simulink model "DockingApproachExample_Ext"  (Simulink 8.7)
settings: Solver=FixedStepDiscrete  StartTime=0.0  StopTime=300  RelTol=1e-3
model workspace (MAT data in the model file):
  input_struct.time = [0; 1; 2; 3; 4; 5; 6; 7; 8; 9; 10; 11; 12; 13; 14; 15; 16; 17; 18; 19; 20; 21; 22; 23; 24; 25; 26; 27; 28; 29; 30; 31; 32; 33; 34; 35; 36; 37; 38; 39; 40; 41; 42; 43; 44; 45; 46; 47; 48; 49; 50; 51; 52; 53; 54; 55; 56; 57; 58; 59; 60; 61; 62; 63; 64; 65; 66; 67; 68; 69; 70; 71; 72; 73; 74; 75; 76; 77; 78; 79; 80; 81; 82; 83; 84; 85; 86; 87; 88; 89; 90; 91; 92; 93; 94; 95; 96; 97; 98; 99; 100]
  input_struct.signals(1).name = 'GroundTrack_OrbitalPosition'
  input_struct.signals(1).values = [82; 91; 13; 92; 64; 10; 28; 55; 96; 97; 16; 98; 96; 49; 81; 15; 43; 92; 80; 96; 66; 4; 85; 94; 68; 76; 75; 40; 66; 18; 71; 4; 28; 5; 10; 83; 70; 32; 96; 4; 44; 39; 77; 80; 19; 49; 45; 65; 71; 76; 28; 68; 66; 17; 12; 50; 96; 35; 59; 23; 76; 26; 51; 70; 90; 96; 55; 14; 15; 26; 85; 26; 82; 25; 93; 35; 20; 26; 62; 48; 36; 84; 59; 55; 92; 29; 76; 76; 39; 57; 8; 6; 54; 78; 94; 13; 57; 47; 2; 34; 17]
  input_struct.signals(1).dimensions = 1
  input_struct.signals(2).name = 'GroundTrack_OrbitalVelocity'
  input_struct.signals(2).values = [80; 32; 53; 17; 61; 27; 66; 69; 75; 46; 9; 23; 92; 16; 83; 54; 100; 8; 45; 11; 97; 1; 78; 82; 87; 9; 40; 26; 81; 44; 92; 19; 27; 15; 14; 87; 58; 55; 15; 86; 63; 36; 52; 41; 8; 24; 13; 19; 24; 42; 5; 91; 95; 50; 49; 34; 91; 37; 12; 79; 39; 25; 41; 10; 14; 95; 96; 58; 6; 24; 36; 83; 2; 5; 17; 65; 74; 65; 46; 55; 30; 75; 19; 69; 19; 37; 63; 79; 9; 93; 78; 49; 44; 45; 31; 51; 52; 82; 80; 65; 38]
  input_struct.signals(2).dimensions = 1
  input_struct.signals(3).name = 'dockVisibility_status'
  input_struct.signals(3).values = [82; 54; 36; 94; 88; 56; 63; 59; 21; 31; 48; 24; 85; 20; 23; 18; 23; 44; 32; 93; 44; 19; 91; 98; 44; 12; 26; 41; 60; 27; 61; 72; 23; 12; 30; 32; 43; 51; 9; 27; 81; 3; 93; 74; 49; 58; 24; 46; 97; 55; 53; 24; 49; 63; 68; 40; 37; 99; 4; 89; 92; 80; 10; 27; 34; 68; 14; 73; 11; 66; 50; 78; 72; 91; 90; 34; 70; 20; 4; 75; 51; 48; 91; 61; 62; 86; 81; 58; 19; 24; 89; 3; 49; 17; 98; 72; 51; 48; 6; 69; 5]
  input_struct.signals(3).dimensions = 1
  input_struct.signals(4).name = 'opticsAvailability_status'
  input_struct.signals(4).values = [1; 1; 1; 1; 1; 1; 1; 1; 1; 1; 1; 1; 1; 1; 1; 1; 1; 1; 1; 1; 1; 1; 1; 1; 1; 1; 1; 1; 1; 1; 1; 1; 1; 1; 1; 1; 1; 1; 1; 1; 1; 1; 1; 1; 1; 1; 1; 1; 1; 1; 1; 1; 1; 1; 1; 1; 1; 1; 1; 1; 1; 1; 1; 1; 1; 1; 1; 1; 1; 1; 1; 1; 1; 1; 1; 1; 1; 1; 1; 1; 1; 1; 1; 1; 1; 1; 1; 1; 1; 1; 1; 1; 1; 1; 1; 1; 1; 1; 1; 1; 1]
  input_struct.signals(4).dimensions = 1
  input_struct.signals(5).name = 'sunlight_status'
  input_struct.signals(5).values = [1; 1; 1; 1; 1; 1; 1; 1; 1; 1; 1; 1; 1; 1; 1; 1; 1; 1; 1; 1; 1; 1; 1; 1; 1; 1; 1; 1; 1; 1; 1; 1; 1; 1; 1; 1; 1; 1; 1; 1; 1; 1; 1; 1; 1; 1; 1; 1; 1; 1; 1; 1; 1; 1; 1; 1; 1; 1; 1; 1; 1; 1; 1; 1; 1; 1; 1; 1; 1; 1; 1; 1; 1; 1; 1; 1; 1; 1; 1; 1; 1; 1; 1; 1; 1; 1; 1; 1; 1; 1; 1; 1; 1; 1; 1; 1; 1; 1; 1; 1; 1]
  input_struct.signals(5).dimensions = 1
  input_struct.signals(6).name = 'GPS_satelliteVisibility_status'
  input_struct.signals(6).values = [12; 94; 65; 48; 64; 55; 65; 55; 73; 53; 100; 22; 11; 11; 7; 41; 45; 37; 77; 63; 78; 94; 98; 20; 14; 70; 10; 53; 54; 87; 49; 40; 68; 75; 53; 35; 15; 59; 27; 5; 76; 25; 45; 69; 36; 74; 40; 69; 71; 45; 2; 34; 43; 28; 20; 83; 43; 89; 40; 77; 40; 81; 76; 38; 22; 80; 95; 33; 68; 44; 84; 77; 17; 87; 99; 52; 89; 59; 16; 20; 41; 75; 83; 79; 32; 54; 9; 12; 14; 68; 50; 19; 50; 15; 6; 86; 57; 93; 70; 59; 82]
  input_struct.signals(6).dimensions = 1
  input_struct.signals(7).name = 'GPS_receiverAvailability_status'
  input_struct.signals(7).values = [1; 1; 1; 1; 1; 1; 1; 1; 1; 1; 1; 1; 1; 1; 1; 1; 1; 1; 1; 1; 1; 1; 1; 1; 1; 1; 1; 1; 1; 1; 1; 1; 1; 1; 1; 1; 1; 1; 1; 1; 1; 1; 1; 1; 1; 1; 1; 1; 1; 1; 1; 1; 1; 1; 1; 1; 1; 1; 1; 1; 1; 1; 1; 1; 1; 1; 1; 1; 1; 1; 1; 1; 1; 1; 1; 1; 1; 1; 1; 1; 1; 1; 1; 1; 1; 1; 1; 1; 1; 1; 1; 1; 1; 1; 1; 1; 1; 1; 1; 1; 1]
  input_struct.signals(7).dimensions = 1
  input_struct.signals(8).name = 'StarPlanetTracker_planetVisibility'
  input_struct.signals(8).values = [34; 90; 12; 99; 54; 71; 100; 29; 42; 47; 77; 82; 11; 18; 36; 6; 53; 34; 18; 21; 91; 68; 47; 92; 11; 75; 74; 57; 19; 60; 30; 14; 22; 90; 8; 25; 6; 45; 2; 90; 20; 10; 31; 46; 11; 100; 34; 30; 7; 30; 5; 51; 77; 64; 9; 9; 78; 91; 54; 11; 83; 34; 30; 75; 2; 5; 67; 61; 53; 73; 71; 79; 29; 70; 56; 40; 7; 79; 34; 61; 75; 11; 13; 55; 49; 90; 80; 74; 6; 8; 9; 80; 95; 69; 14; 73; 12; 12; 65; 33; 66]
  input_struct.signals(8).dimensions = 1
  input_struct.signals(9).name = 'StarPlanetTracker_starVisibility'
  input_struct.signals(9).values = [75; 59; 75; 24; 74; 98; 87; 9; 37; 37; 69; 60; 79; 37; 21; 9; 78; 21; 39; 56; 23; 65; 49; 16; 79; 11; 30; 24; 54; 10; 41; 11; 12; 79; 30; 61; 97; 44; 70; 76; 44; 66; 11; 94; 19; 27; 80; 49; 77; 40; 28; 4; 68; 43; 46; 61; 6; 32; 78; 70; 13; 14; 10; 1; 43; 66; 73; 54; 11; 64; 13; 14; 10; 15; 17; 20; 32; 32; 22; 26; 90; 71; 56; 19; 22; 8; 92; 71; 56; 32; 17; 63; 99; 18; 26; 40; 8; 69; 41; 99; 41]
  input_struct.signals(9).dimensions = 1
  input_struct.signals(10).name = 'InertialNavigation_time'
  input_struct.signals(10).values = [1; 1; 1; 1; 1; 1; 1; 1; 1; 1; 1; 1; 1; 1; 1; 1; 1; 1; 1; 1; 1; 1; 1; 1; 1; 1; 1; 1; 1; 1; 1; 1; 1; 1; 1; 1; 1; 1; 1; 1; 1; 1; 1; 1; 1; 1; 1; 1; 1; 1; 1; 1; 1; 1; 1; 1; 1; 1; 1; 1; 1; 1; 1; 1; 1; 1; 1; 1; 1; 1; 1; 1; 1; 1; 1; 1; 1; 1; 1; 1; 1; 1; 1; 1; 1; 1; 1; 1; 1; 1; 1; 1; 1; 1; 1; 1; 1; 1; 1; 1; 1]
  input_struct.signals(10).dimensions = 1
  input_struct.signals(11).name = 'GroundTrack_Time'
  input_struct.signals(11).values = [19; 73; 38; 85; 74; 58; 18; 96; 27; 93; 23; 38; 9; 65; 19; 5; 73; 35; 67; 39; 63; 3; 92; 81; 75; 82; 39; 62; 58; 54; 28; 25; 46; 23; 81; 99; 3; 54; 9; 81; 99; 7; 94; 2; 69; 79; 54; 89; 90; 63; 14; 22; 19; 5; 11; 62; 94; 36; 42; 99; 95; 68; 99; 77; 34; 67; 25; 30; 69; 53; 42; 61; 76; 59; 56; 59; 52; 9; 72; 100; 36; 98; 35; 89; 46; 42; 22; 13; 31; 73; 79; 70; 1; 85; 93; 78; 5; 38; 71; 73; 23]
  input_struct.signals(11).dimensions = 1
  input_struct.signals(12).name = 'RealTimeClock_time'
  input_struct.signals(12).values = [27; 68; 48; 63; 24; 18; 83; 77; 94; 11; 19; 10; 49; 20; 90; 10; 5; 56; 78; 32; 18; 34; 22; 52; 91; 63; 11; 40; 6; 51; 44; 100; 82; 49; 90; 14; 40; 93; 92; 72; 62; 35; 94; 13; 74; 65; 84; 40; 75; 84; 33; 56; 98; 55; 34; 62; 37; 76; 42; 50; 70; 98; 33; 84; 74; 96; 4; 36; 67; 29; 24; 72; 63; 60; 67; 5; 35; 46; 25; 72; 86; 29; 74; 14; 84; 14; 59; 37; 81; 51; 49; 88; 36; 45; 97; 5; 98; 19; 67; 59; 68]
  input_struct.signals(12).dimensions = 1
  input_struct.signals(13).name = 'StageTransition'
  input_struct.signals(13).values = [37; 63; 82; 2; 9; 98; 66; 24; 41; 13; 27; 26; 34; 16; 35; 13; 89; 10; 94; 40; 5; 35; 74; 80; 55; 69; 90; 6; 31; 5; 20; 73; 73; 88; 59; 8; 93; 81; 29; 55; 99; 72; 84; 44; 48; 57; 27; 75; 51; 65; 31; 14; 48; 37; 79; 79; 67; 14; 3; 56; 31; 94; 99; 29; 81; 90; 60; 89; 95; 55; 73; 58; 3; 45; 65; 53; 38; 94; 83; 85; 38; 60; 88; 94; 67; 21; 66; 8; 41; 67; 94; 82; 49; 76; 42; 98; 99; 87; 39; 46; 25]
  input_struct.signals(13).dimensions : numeric (value not decoded)
libraries: simulink x11
(part 1 of 2)
settings Model: Creator=mwwhalen  LastModifiedBy=bourbouh
settings DataIOCC: ExternalInput=[t,u]  SaveFormat=Dataset  SignalLoggingSaveFormat=ModelDataLogs
settings OptimizationCC: ExpressionDepthLimit=2147483647  InitFltsAndDblsToZero=on
settings DebuggingCC: SaveWithParameterizedLinksMsg=none  SignalResolutionControl=TryResolveAllWithWarning  SolverPrmCheckMsg=warning  MultiTaskDSMMsg=warning  MultiTaskCondExecSysMsg=none  FcnCallInpInsideContextMsg=UseLocalSettings  StateNameClashWarn=warning
settings SFSimCC: SimParseCustomCode=off
settings RTWCC: PackageGeneratedCodeAndArtifacts=on  PackageName=DockingApproachExample_Ext_Code.zip  RTWCompilerOptimization=on
settings GRTTargetCC: TargetFcnLib=ansi_tfl_tmw.mat  CombineOutputUpdateFcns=off  GRTInterface=on

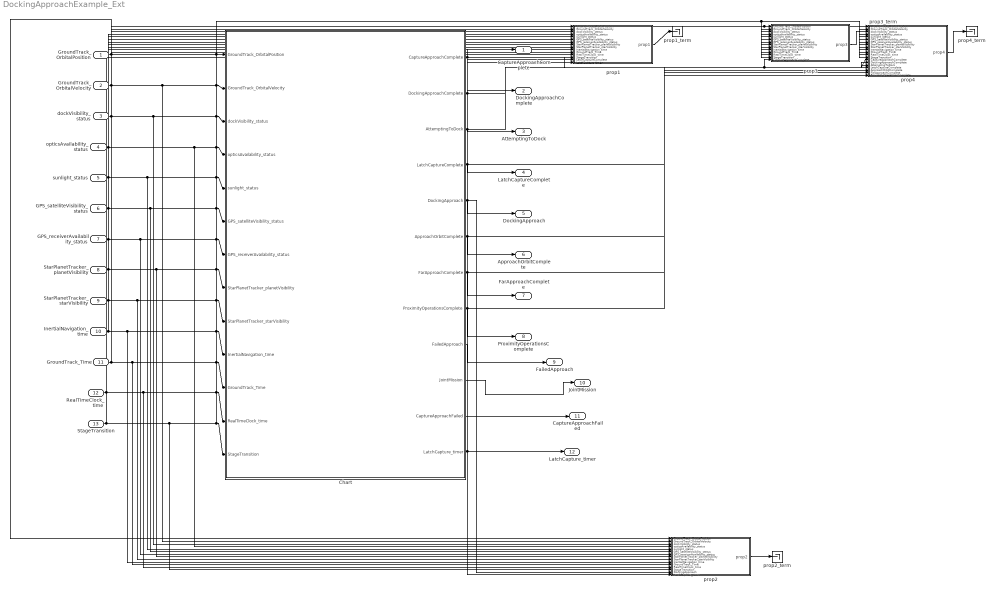
== system DockingApproachExample_Ext ==
  GroundTrack_OrbitalPosition : Inport
  GroundTrack_OrbitalVelocity : Inport  Port=2
  dockVisibility_status : Inport  Port=3
  opticsAvailability_status : Inport  Port=4
  sunlight_status : Inport  Port=5
  GPS_satelliteVisibility_status : Inport  Port=6
  GPS_receiverAvailability_status : Inport  Port=7
  StarPlanetTracker_planetVisibility : Inport  Port=8
  StarPlanetTracker_starVisibility : Inport  Port=9
  InertialNavigation_time : Inport  Port=10
  GroundTrack_Time : Inport  Port=11
  RealTimeClock_time : Inport  Port=12
  StageTransition : Inport  Port=13
  Chart : Stateflow chart  TreatAsAtomicUnit=on
  prop1 : Subsystem  TreatAsAtomicUnit=on  mask(Observer){AnnotationType=ensures, ObserverType=[]}
      mask prompts: AnnotationType "Type of annotation (pre/post...)"; ObserverType "Observer type"
      mask help:
      | Set an observer for the system.
      | The annotation type parameter sets the type of observer:
      | - requires : pre-condition
      | - ensures : post-condition
      | - assert : an assertion
      | - observer : the observer computes a special type of properties
      mask TypeOptions AnnotationType: ensures | requires | assert | observer
      mask Callback AnnotationType:
      | paramStr = get_param(gcb, 'MaskValues');
      | if strcmp(paramStr{1}(1),'o')
      | set_param(gcb,'MaskVisibilities',{'on';'on'});
      | paramStr{2} = 'ellipsoid';
      | set_param(gcb,'MaskValues',paramStr);
      | else
      | set_param(gcb,'MaskVisibilities',{'on';'off'});
      | end
      | clear paramStr;
      mask Callback ObserverType:
      | paramStr = get_param(gcb, 'MaskValues');
      | if strcmp(paramStr{1}(1),'o')
      | set_param(gcb,'MaskVisibilities',{'on';'on'});
      | paramStr{2} = 'ellipsoid';
      | set_param(gcb,'MaskValues',paramStr);
      | else
      | set_param(gcb,'MaskVisibilities',{'on';'off'});
      | end
      | clear paramStr;
      mask Display:
      | color('black')
      | text(0.5, 0.5, ['Property: ''' get_param(gcb,'name') ''''], 'horizontalAlignment', 'center');
      | text(0.99, 0.03, '{\bf\fontsize{12}SAFE}', 'hor', 'right', 'ver', 'bottom', 'texmode', 'on');
  prop1_term : Terminator
  prop2 : Subsystem  TreatAsAtomicUnit=on  mask(Observer){AnnotationType=ensures, ObserverType=[]}
      mask prompts: AnnotationType "Type of annotation (pre/post...)"; ObserverType "Observer type"
      mask help:
      | Set an observer for the system.
      | The annotation type parameter sets the type of observer:
      | - requires : pre-condition
      | - ensures : post-condition
      | - assert : an assertion
      | - observer : the observer computes a special type of properties
      mask TypeOptions AnnotationType: ensures | requires | assert | observer
      mask Callback AnnotationType:
      | paramStr = get_param(gcb, 'MaskValues');
      | if strcmp(paramStr{1}(1),'o')
      | set_param(gcb,'MaskVisibilities',{'on';'on'});
      | paramStr{2} = 'ellipsoid';
      | set_param(gcb,'MaskValues',paramStr);
      | else
      | set_param(gcb,'MaskVisibilities',{'on';'off'});
      | end
      | clear paramStr;
      mask Callback ObserverType:
      | paramStr = get_param(gcb, 'MaskValues');
      | if strcmp(paramStr{1}(1),'o')
      | set_param(gcb,'MaskVisibilities',{'on';'on'});
      | paramStr{2} = 'ellipsoid';
      | set_param(gcb,'MaskValues',paramStr);
      | else
      | set_param(gcb,'MaskVisibilities',{'on';'off'});
      | end
      | clear paramStr;
      mask Display:
      | color('black')
      | text(0.5, 0.5, ['Property: ''' get_param(gcb,'name') ''''], 'horizontalAlignment', 'center');
      | text(0.99, 0.03, '{\bf\fontsize{12}SAFE}', 'hor', 'right', 'ver', 'bottom', 'texmode', 'on');
  prop2_term : Terminator
  prop3 : Subsystem  TreatAsAtomicUnit=on  mask(Observer){AnnotationType=ensures, ObserverType=[]}
      mask prompts: AnnotationType "Type of annotation (pre/post...)"; ObserverType "Observer type"
      mask help:
      | Set an observer for the system.
      | The annotation type parameter sets the type of observer:
      | - requires : pre-condition
      | - ensures : post-condition
      | - assert : an assertion
      | - observer : the observer computes a special type of properties
      mask TypeOptions AnnotationType: ensures | requires | assert | observer
      mask Callback AnnotationType:
      | paramStr = get_param(gcb, 'MaskValues');
      | if strcmp(paramStr{1}(1),'o')
      | set_param(gcb,'MaskVisibilities',{'on';'on'});
      | paramStr{2} = 'ellipsoid';
      | set_param(gcb,'MaskValues',paramStr);
      | else
      | set_param(gcb,'MaskVisibilities',{'on';'off'});
      | end
      | clear paramStr;
      mask Callback ObserverType:
      | paramStr = get_param(gcb, 'MaskValues');
      | if strcmp(paramStr{1}(1),'o')
      | set_param(gcb,'MaskVisibilities',{'on';'on'});
      | paramStr{2} = 'ellipsoid';
      | set_param(gcb,'MaskValues',paramStr);
      | else
      | set_param(gcb,'MaskVisibilities',{'on';'off'});
      | end
      | clear paramStr;
      mask Display:
      | color('black')
      | text(0.5, 0.5, ['Property: ''' get_param(gcb,'name') ''''], 'horizontalAlignment', 'center');
      | text(0.99, 0.03, '{\bf\fontsize{12}SAFE}', 'hor', 'right', 'ver', 'bottom', 'texmode', 'on');
  prop3_term : Terminator
  prop4 : Subsystem  TreatAsAtomicUnit=on  mask(Observer){AnnotationType=ensures, ObserverType=[]}
      mask prompts: AnnotationType "Type of annotation (pre/post...)"; ObserverType "Observer type"
      mask help:
      | Set an observer for the system.
      | The annotation type parameter sets the type of observer:
      | - requires : pre-condition
      | - ensures : post-condition
      | - assert : an assertion
      | - observer : the observer computes a special type of properties
      mask TypeOptions AnnotationType: ensures | requires | assert | observer
      mask Callback AnnotationType:
      | paramStr = get_param(gcb, 'MaskValues');
      | if strcmp(paramStr{1}(1),'o')
      | set_param(gcb,'MaskVisibilities',{'on';'on'});
      | paramStr{2} = 'ellipsoid';
      | set_param(gcb,'MaskValues',paramStr);
      | else
      | set_param(gcb,'MaskVisibilities',{'on';'off'});
      | end
      | clear paramStr;
      mask Callback ObserverType:
      | paramStr = get_param(gcb, 'MaskValues');
      | if strcmp(paramStr{1}(1),'o')
      | set_param(gcb,'MaskVisibilities',{'on';'on'});
      | paramStr{2} = 'ellipsoid';
      | set_param(gcb,'MaskValues',paramStr);
      | else
      | set_param(gcb,'MaskVisibilities',{'on';'off'});
      | end
      | clear paramStr;
      mask Display:
      | color('black')
      | text(0.5, 0.5, ['Property: ''' get_param(gcb,'name') ''''], 'horizontalAlignment', 'center');
      | text(0.99, 0.03, '{\bf\fontsize{12}TIMEOUT}', 'hor', 'right', 'ver', 'bottom', 'texmode', 'on');
  prop4_term : Terminator
  CaptureApproachComplete : Outport
  DockingApproachComplete : Outport  Port=2
  AttemptingToDock : Outport  Port=3
  LatchCaptureComplete : Outport  Port=4
  DockingApproach : Outport  Port=5
  ApproachOrbitComplete : Outport  Port=6
  FarApproachComplete : Outport  Port=7
  ProximityOperationsComplete : Outport  Port=8
  FailedApproach : Outport  Port=9
  JointMission : Outport  Port=10
  CaptureApproachFailed : Outport  Port=11
  LatchCapture_timer : Outport  Port=12
  wires:
  GroundTrack_OrbitalVelocity/1 -> prop3/2(GroundTrack_OrbitalVelocity), prop4/2(GroundTrack_OrbitalVelocity), Chart/2(GroundTrack_OrbitalVelocity), prop2/2(GroundTrack_OrbitalVelocity), prop1/2(GroundTrack_OrbitalVelocity)
  dockVisibility_status/1 -> prop3/3(dockVisibility_status), prop4/3(dockVisibility_status), Chart/3(dockVisibility_status), prop2/3(dockVisibility_status), prop1/3(dockVisibility_status)
  opticsAvailability_status/1 -> prop3/4(opticsAvailability_status), prop4/4(opticsAvailability_status), Chart/4(opticsAvailability_status), prop2/4(opticsAvailability_status), prop1/4(opticsAvailability_status)
  sunlight_status/1 -> prop3/5(sunlight_status), prop4/5(sunlight_status), Chart/5(sunlight_status), prop2/5(sunlight_status), prop1/5(sunlight_status)
  GPS_satelliteVisibility_status/1 -> prop3/6(GPS_satelliteVisibility_status), prop4/6(GPS_satelliteVisibility_status), Chart/6(GPS_satelliteVisibility_status), prop2/6(GPS_satelliteVisibility_status), prop1/6(GPS_satelliteVisibility_status)
  StarPlanetTracker_planetVisibility/1 -> prop3/8(StarPlanetTracker_planetVisibility), prop4/8(StarPlanetTracker_planetVisibility), Chart/8(StarPlanetTracker_planetVisibility), prop2/8(StarPlanetTracker_planetVisibility), prop1/8(StarPlanetTracker_planetVisibility)
  StarPlanetTracker_starVisibility/1 -> prop3/9(StarPlanetTracker_starVisibility), prop4/9(StarPlanetTracker_starVisibility), Chart/9(StarPlanetTracker_starVisibility), prop2/9(StarPlanetTracker_starVisibility), prop1/9(StarPlanetTracker_starVisibility)
  InertialNavigation_time/1 -> prop3/10(InertialNavigation_time), prop4/10(InertialNavigation_time), Chart/10(InertialNavigation_time), prop2/10(InertialNavigation_time), prop1/10(InertialNavigation_time)
  GroundTrack_Time/1 -> prop3/11(GroundTrack_Time), prop4/11(GroundTrack_Time), Chart/11(GroundTrack_Time), prop2/11(GroundTrack_Time), prop1/11(GroundTrack_Time)
  RealTimeClock_time/1 -> prop3/12(RealTimeClock_time), prop4/12(RealTimeClock_time), Chart/12(RealTimeClock_time), prop2/12(RealTimeClock_time), prop1/12(RealTimeClock_time)
  GroundTrack_OrbitalPosition/1 -> prop3/1(GroundTrack_OrbitalPosition), prop4/1(GroundTrack_OrbitalPosition), Chart/1(GroundTrack_OrbitalPosition), prop1/1(GroundTrack_OrbitalPosition), prop2/1(GroundTrack_OrbitalPosition)
  StageTransition/1 -> prop3/13(StageTransition), prop4/13(StageTransition), Chart/13(StageTransition), prop2/13(StageTransition), prop1/13(StageTransition)
  GPS_receiverAvailability_status/1 -> prop3/7(GPS_receiverAvailability_status), prop4/7(GPS_receiverAvailability_status), Chart/7(GPS_receiverAvailability_status), prop2/7(GPS_receiverAvailability_status), prop1/7(GPS_receiverAvailability_status)
  Chart/2(DockingApproachComplete) -> DockingApproachComplete/1, prop4/15(DockingApproachComplete)
  Chart/1(CaptureApproachComplete) -> prop3/14(CaptureApproachComplete), prop4/14(CaptureApproachComplete), CaptureApproachComplete/1
  Chart/3(AttemptingToDock) -> AttemptingToDock/1, prop4/16(AttemptingToDock)
  Chart/4(LatchCaptureComplete) -> LatchCaptureComplete/1, prop1/14(LatchCaptureComplete), prop4/17(LatchCaptureComplete)
  Chart/5(DockingApproach) -> DockingApproach/1, prop2/14(DockingApproach)
  Chart/6(ApproachOrbitComplete) -> ApproachOrbitComplete/1, prop4/18(ApproachOrbitComplete)
  Chart/7(FarApproachComplete) -> FarApproachComplete/1, prop4/19(FarApproachComplete)
  Chart/8(ProximityOperationsComplete) -> ProximityOperationsComplete/1, prop4/20(ProximityOperationsComplete)
  Chart/9(FailedApproach) -> FailedApproach/1
  Chart/10(JointMission) -> JointMission/1
  Chart/11(CaptureApproachFailed) -> CaptureApproachFailed/1
  Chart/12(LatchCapture_timer) -> LatchCapture_timer/1, prop1/15(LatchCapture_timer), prop2/15(LatchCapture_timer)
  prop1/1(prop1) -> prop1_term/1
  prop2/1(prop2) -> prop2_term/1
  prop3/1(prop3) -> prop3_term/1
  prop4/1(prop4) -> prop4_term/1

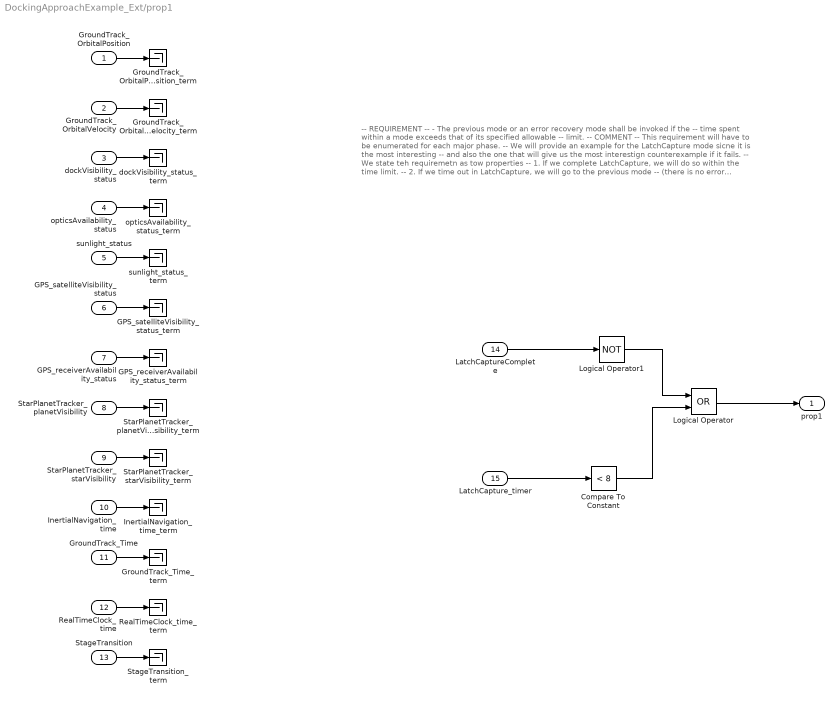
== system DockingApproachExample_Ext/prop1 ==
  note: -- REQUIREMENT
      | -- - The previous mode or an error recovery mode shall be invoked if the
      | -- time spent within a mode exceeds that of its specified allowable
      | -- limit.
      |
      | -- COMMENT
      | -- This requirement will have to be enumerated for each major phase.
      | -- We will provide an example for the LatchCapture mode sicne it is the most interesting
      | -- and also the one that will give us the most interestign counterexample if it fails.
      | -- We state teh requiremetn as tow properties
      | -- 1. If we complete LatchCapture, we will do so within the time limit.
      | -- 2. If we time out in LatchCapture, we will go to the previous mode
      | -- (there is no error recovery mode in the model we were given).
      |
      | -- 1
      | INVARSPEC ((LatchCaptureComplete = 1) ->
      | (LatchCapture_timer < LatchCapture_timer_upper_limit))
  GroundTrack_OrbitalPosition : Inport
  GroundTrack_OrbitalVelocity : Inport  Port=2
  dockVisibility_status : Inport  Port=3
  opticsAvailability_status : Inport  Port=4
  sunlight_status : Inport  Port=5
  GPS_satelliteVisibility_status : Inport  Port=6
  GPS_receiverAvailability_status : Inport  Port=7
  StarPlanetTracker_planetVisibility : Inport  Port=8
  StarPlanetTracker_starVisibility : Inport  Port=9
  InertialNavigation_time : Inport  Port=10
  GroundTrack_Time : Inport  Port=11
  RealTimeClock_time : Inport  Port=12
  StageTransition : Inport  Port=13
  LatchCaptureComplete : Inport  Port=14
  LatchCapture_timer : Inport  Port=15
  Compare To Constant : simulink/Logic and Bit Operations/Compare To Constant  relop=<  const=8  OutDataTypeStr=boolean
  GPS_receiverAvailability_status_term : Terminator
  GPS_satelliteVisibility_status_term : Terminator
  GroundTrack_OrbitalPosition_term : Terminator
  GroundTrack_OrbitalVelocity_term : Terminator
  GroundTrack_Time_term : Terminator
  InertialNavigation_time_term : Terminator
  Logical Operator : Logic  Operator=OR  AllPortsSameDT=off  OutDataTypeStr=boolean
  Logical Operator1 : Logic  Operator=NOT  AllPortsSameDT=off  OutDataTypeStr=boolean
  RealTimeClock_time_term : Terminator
  StageTransition_term : Terminator
  StarPlanetTracker_planetVisibility_term : Terminator
  StarPlanetTracker_starVisibility_term : Terminator
  dockVisibility_status_term : Terminator
  opticsAvailability_status_term : Terminator
  sunlight_status_term : Terminator
  prop1 : Outport
  wires:
  GroundTrack_OrbitalPosition/1 -> GroundTrack_OrbitalPosition_term/1
  GroundTrack_OrbitalVelocity/1 -> GroundTrack_OrbitalVelocity_term/1
  dockVisibility_status/1 -> dockVisibility_status_term/1
  opticsAvailability_status/1 -> opticsAvailability_status_term/1
  sunlight_status/1 -> sunlight_status_term/1
  GPS_satelliteVisibility_status/1 -> GPS_satelliteVisibility_status_term/1
  GPS_receiverAvailability_status/1 -> GPS_receiverAvailability_status_term/1
  StarPlanetTracker_planetVisibility/1 -> StarPlanetTracker_planetVisibility_term/1
  StarPlanetTracker_starVisibility/1 -> StarPlanetTracker_starVisibility_term/1
  InertialNavigation_time/1 -> InertialNavigation_time_term/1
  GroundTrack_Time/1 -> GroundTrack_Time_term/1
  RealTimeClock_time/1 -> RealTimeClock_time_term/1
  StageTransition/1 -> StageTransition_term/1
  LatchCaptureComplete/1 -> Logical Operator1/1
  LatchCapture_timer/1 -> Compare To Constant/1
  Logical Operator1/1 -> Logical Operator/1
  Compare To Constant/1 -> Logical Operator/2
  Logical Operator/1 -> prop1/1

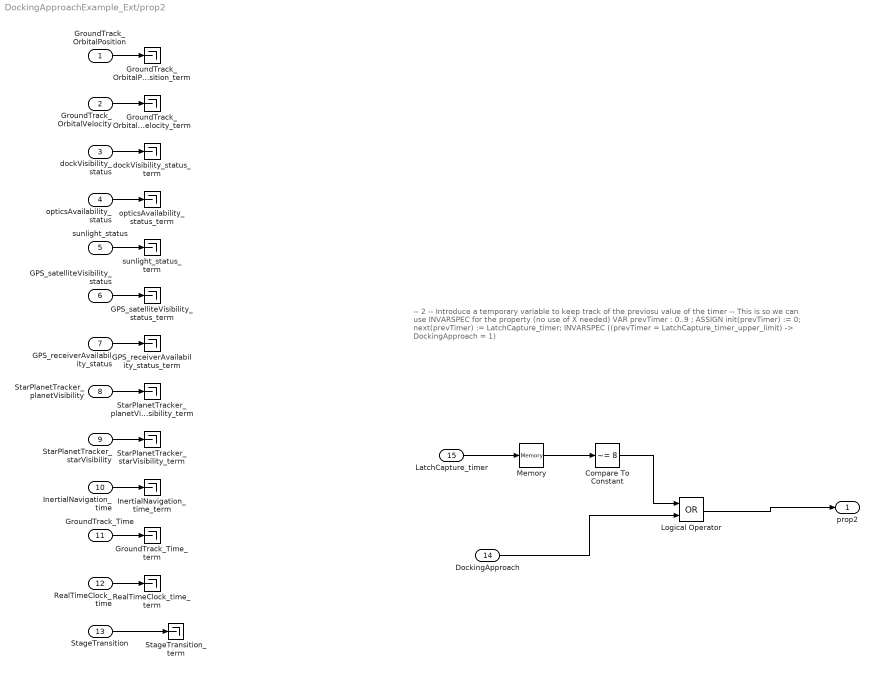
== system DockingApproachExample_Ext/prop2 ==
  note: -- 2
      | -- Introduce a temporary variable to keep track of the previosu value of the timer
      | -- This is so we can use INVARSPEC for the property (no use of X needed)
      | VAR
      | prevTimer : 0..9 ;
      | ASSIGN
      | init(prevTimer) := 0;
      | next(prevTimer) := LatchCapture_timer;
      |
      | INVARSPEC ((prevTimer = LatchCapture_timer_upper_limit) -> DockingApproach = 1)
  GroundTrack_OrbitalPosition : Inport
  GroundTrack_OrbitalVelocity : Inport  Port=2
  dockVisibility_status : Inport  Port=3
  opticsAvailability_status : Inport  Port=4
  sunlight_status : Inport  Port=5
  GPS_satelliteVisibility_status : Inport  Port=6
  GPS_receiverAvailability_status : Inport  Port=7
  StarPlanetTracker_planetVisibility : Inport  Port=8
  StarPlanetTracker_starVisibility : Inport  Port=9
  InertialNavigation_time : Inport  Port=10
  GroundTrack_Time : Inport  Port=11
  RealTimeClock_time : Inport  Port=12
  StageTransition : Inport  Port=13
  DockingApproach : Inport  Port=14
  LatchCapture_timer : Inport  Port=15
  Compare To Constant : simulink/Logic and Bit Operations/Compare To Constant  relop=~=  const=8  OutDataTypeStr=boolean
  GPS_receiverAvailability_status_term : Terminator
  GPS_satelliteVisibility_status_term : Terminator
  GroundTrack_OrbitalPosition_term : Terminator
  GroundTrack_OrbitalVelocity_term : Terminator
  GroundTrack_Time_term : Terminator
  InertialNavigation_time_term : Terminator
  Logical Operator : Logic  Operator=OR  AllPortsSameDT=off  OutDataTypeStr=boolean
  Memory : Memory
  RealTimeClock_time_term : Terminator
  StageTransition_term : Terminator
  StarPlanetTracker_planetVisibility_term : Terminator
  StarPlanetTracker_starVisibility_term : Terminator
  dockVisibility_status_term : Terminator
  opticsAvailability_status_term : Terminator
  sunlight_status_term : Terminator
  prop2 : Outport
  wires:
  GroundTrack_OrbitalPosition/1 -> GroundTrack_OrbitalPosition_term/1
  GroundTrack_OrbitalVelocity/1 -> GroundTrack_OrbitalVelocity_term/1
  dockVisibility_status/1 -> dockVisibility_status_term/1
  opticsAvailability_status/1 -> opticsAvailability_status_term/1
  sunlight_status/1 -> sunlight_status_term/1
  GPS_satelliteVisibility_status/1 -> GPS_satelliteVisibility_status_term/1
  GPS_receiverAvailability_status/1 -> GPS_receiverAvailability_status_term/1
  StarPlanetTracker_planetVisibility/1 -> StarPlanetTracker_planetVisibility_term/1
  StarPlanetTracker_starVisibility/1 -> StarPlanetTracker_starVisibility_term/1
  InertialNavigation_time/1 -> InertialNavigation_time_term/1
  GroundTrack_Time/1 -> GroundTrack_Time_term/1
  RealTimeClock_time/1 -> RealTimeClock_time_term/1
  StageTransition/1 -> StageTransition_term/1
  DockingApproach/1 -> Logical Operator/2
  LatchCapture_timer/1 -> Memory/1
  Memory/1 -> Compare To Constant/1
  Compare To Constant/1 -> Logical Operator/1
  Logical Operator/1 -> prop2/1

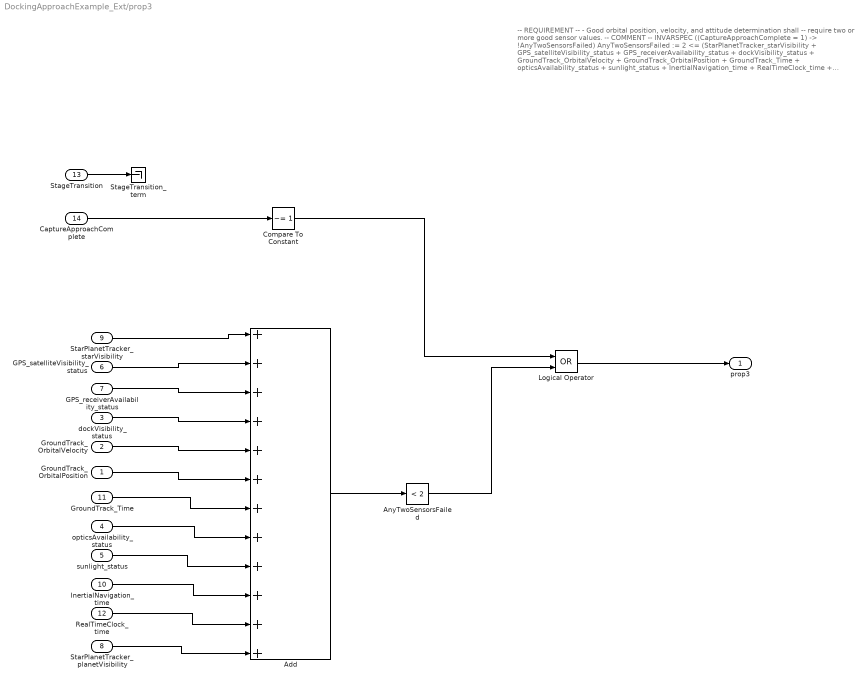
== system DockingApproachExample_Ext/prop3 ==
  note: -- REQUIREMENT
      | -- - Good orbital position, velocity, and attitude determination shall
      | -- require two or more good sensor values.
      |
      | -- COMMENT
      | --
      |
      | INVARSPEC ((CaptureApproachComplete = 1) -> !AnyTwoSensorsFailed)
      |
      | AnyTwoSensorsFailed := 2 <= (StarPlanetTracker_starVisibility +
      | GPS_satelliteVisibility_status +
      | GPS_receiverAvailability_status +
      | dockVisibility_status +
      | GroundTrack_OrbitalVelocity +
      | GroundTrack_OrbitalPosition +
      | GroundTrack_Time +
      | opticsAvailability_status +
      | sunlight_status +
      | InertialNavigation_time +
      | RealTimeClock_time +
      | StarPlanetTracker_planetVisibility );
  GroundTrack_OrbitalPosition : Inport
  GroundTrack_OrbitalVelocity : Inport  Port=2
  dockVisibility_status : Inport  Port=3
  opticsAvailability_status : Inport  Port=4
  sunlight_status : Inport  Port=5
  GPS_satelliteVisibility_status : Inport  Port=6
  GPS_receiverAvailability_status : Inport  Port=7
  StarPlanetTracker_planetVisibility : Inport  Port=8
  StarPlanetTracker_starVisibility : Inport  Port=9
  InertialNavigation_time : Inport  Port=10
  GroundTrack_Time : Inport  Port=11
  RealTimeClock_time : Inport  Port=12
  StageTransition : Inport  Port=13
  CaptureApproachComplete : Inport  Port=14
  Add : Sum  Inputs=++++++++++++  AccumDataTypeStr=int8  OutDataTypeStr=int8
  AnyTwoSensorsFailed : simulink/Logic and Bit Operations/Compare To Constant  relop=<  const=2  OutDataTypeStr=boolean
  Compare To Constant : simulink/Logic and Bit Operations/Compare To Constant  relop=~=  const=1  OutDataTypeStr=boolean
  Logical Operator : Logic  Operator=OR  AllPortsSameDT=off  OutDataTypeStr=boolean
  StageTransition_term : Terminator
  prop3 : Outport
  wires:
  GroundTrack_OrbitalPosition/1 -> Add/6
  GroundTrack_OrbitalVelocity/1 -> Add/5
  dockVisibility_status/1 -> Add/4
  opticsAvailability_status/1 -> Add/8
  sunlight_status/1 -> Add/9
  GPS_satelliteVisibility_status/1 -> Add/2
  GPS_receiverAvailability_status/1 -> Add/3
  StarPlanetTracker_planetVisibility/1 -> Add/12
  StarPlanetTracker_starVisibility/1 -> Add/1
  InertialNavigation_time/1 -> Add/10
  GroundTrack_Time/1 -> Add/7
  RealTimeClock_time/1 -> Add/11
  StageTransition/1 -> StageTransition_term/1
  CaptureApproachComplete/1 -> Compare To Constant/1
  Add/1 -> AnyTwoSensorsFailed/1
  Compare To Constant/1 -> Logical Operator/1
  AnyTwoSensorsFailed/1 -> Logical Operator/2
  Logical Operator/1 -> prop3/1

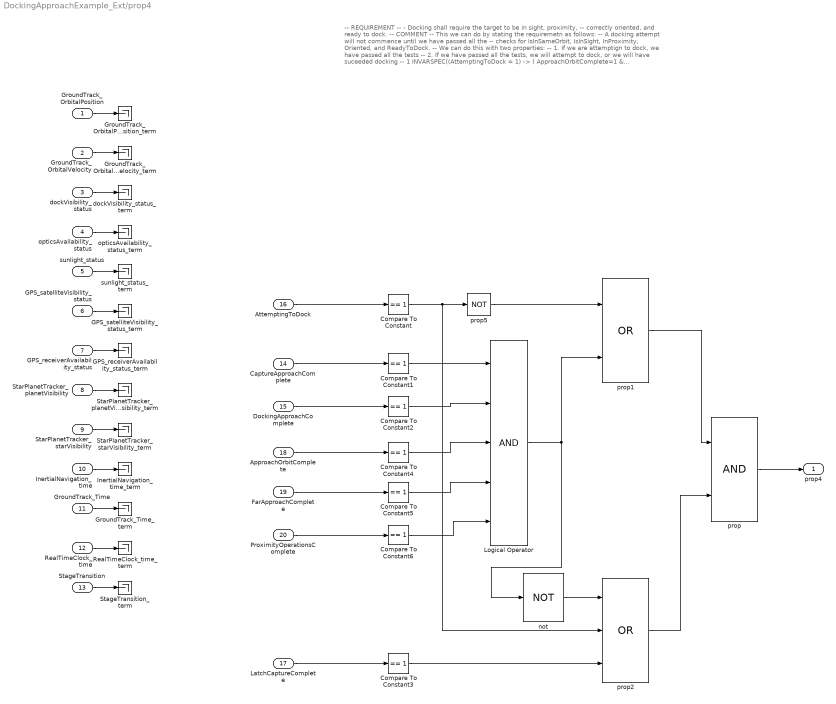
== system DockingApproachExample_Ext/prop4 ==
  note: -- REQUIREMENT
      | -- - Docking shall require the target to be in sight, proximity,
      | -- correctly oriented, and ready to dock.
      |
      | -- COMMENT
      | -- This we can do by stating the requiremetn as follows:
      | -- A docking attempt will not commence until we have passed all the
      | -- checks for IsInSameOrbit, IsInSight, InProximity, Oriented, and ReadyToDock.
      | -- We can do this with two properties:
      | -- 1. If we are attemptign to dock, we have passed all the tests
      | -- 2. If we have passed all the tests, we will attempt to dock, or we will have suceeded docking
      |
      | -- 1
      | INVARSPEC((AttemptingToDock = 1) ->
      | ( ApproachOrbitComplete=1 &
      | ProximityOperationsComplete=1 &
      | FarApproachComplete=1 &
      | CaptureApproachComplete= 1 &
      | DockingApproachComplete= 1 ))
      | -- 2
      | INVARSPEC ( ( ( ApproachOrbitComplete=1 &
      | ProximityOperationsComplete=1 &
      | FarApproachComplete=1 &
      | CaptureApproachComplete= 1 &
      | DockingApproachComplete= 1 ) -> (AttemptingToDock = 1) )
      | |
      | (LatchCaptureComplete = 1) )
  GroundTrack_OrbitalPosition : Inport
  GroundTrack_OrbitalVelocity : Inport  Port=2
  dockVisibility_status : Inport  Port=3
  opticsAvailability_status : Inport  Port=4
  sunlight_status : Inport  Port=5
  GPS_satelliteVisibility_status : Inport  Port=6
  GPS_receiverAvailability_status : Inport  Port=7
  StarPlanetTracker_planetVisibility : Inport  Port=8
  StarPlanetTracker_starVisibility : Inport  Port=9
  InertialNavigation_time : Inport  Port=10
  GroundTrack_Time : Inport  Port=11
  RealTimeClock_time : Inport  Port=12
  StageTransition : Inport  Port=13
  CaptureApproachComplete : Inport  Port=14
  DockingApproachComplete : Inport  Port=15
  AttemptingToDock : Inport  Port=16
  LatchCaptureComplete : Inport  Port=17
  ApproachOrbitComplete : Inport  Port=18
  FarApproachComplete : Inport  Port=19
  ProximityOperationsComplete : Inport  Port=20
  Compare To Constant{,1..6} (7 alike) : simulink/Logic and Bit Operations/Compare To Constant  relop===  const=1  OutDataTypeStr=boolean
  GPS_receiverAvailability_status_term : Terminator
  GPS_satelliteVisibility_status_term : Terminator
  GroundTrack_OrbitalPosition_term : Terminator
  GroundTrack_OrbitalVelocity_term : Terminator
  GroundTrack_Time_term : Terminator
  InertialNavigation_time_term : Terminator
  Logical Operator : Logic  Inputs=5  AllPortsSameDT=off  OutDataTypeStr=boolean
  RealTimeClock_time_term : Terminator
  StageTransition_term : Terminator
  StarPlanetTracker_planetVisibility_term : Terminator
  StarPlanetTracker_starVisibility_term : Terminator
  dockVisibility_status_term : Terminator
  not : Logic  Operator=NOT  AllPortsSameDT=off  OutDataTypeStr=boolean
  opticsAvailability_status_term : Terminator
  prop : Logic  AllPortsSameDT=off  OutDataTypeStr=boolean
  prop1 : Logic  Operator=OR  AllPortsSameDT=off  OutDataTypeStr=boolean
  prop2 : Logic  Operator=OR  Inputs=3  AllPortsSameDT=off  OutDataTypeStr=boolean
  prop5 : Logic  Operator=NOT  AllPortsSameDT=off  OutDataTypeStr=boolean
  sunlight_status_term : Terminator
  prop4 : Outport
  wires:
  GroundTrack_OrbitalPosition/1 -> GroundTrack_OrbitalPosition_term/1
  GroundTrack_OrbitalVelocity/1 -> GroundTrack_OrbitalVelocity_term/1
  dockVisibility_status/1 -> dockVisibility_status_term/1
  opticsAvailability_status/1 -> opticsAvailability_status_term/1
  sunlight_status/1 -> sunlight_status_term/1
  GPS_satelliteVisibility_status/1 -> GPS_satelliteVisibility_status_term/1
  GPS_receiverAvailability_status/1 -> GPS_receiverAvailability_status_term/1
  StarPlanetTracker_planetVisibility/1 -> StarPlanetTracker_planetVisibility_term/1
  StarPlanetTracker_starVisibility/1 -> StarPlanetTracker_starVisibility_term/1
  InertialNavigation_time/1 -> InertialNavigation_time_term/1
  GroundTrack_Time/1 -> GroundTrack_Time_term/1
  RealTimeClock_time/1 -> RealTimeClock_time_term/1
  StageTransition/1 -> StageTransition_term/1
  AttemptingToDock/1 -> Compare To Constant/1
  CaptureApproachComplete/1 -> Compare To Constant1/1
  ProximityOperationsComplete/1 -> Compare To Constant6/1
  FarApproachComplete/1 -> Compare To Constant5/1
  ApproachOrbitComplete/1 -> Compare To Constant4/1
  LatchCaptureComplete/1 -> Compare To Constant3/1
  DockingApproachComplete/1 -> Compare To Constant2/1
  Compare To Constant6/1 -> Logical Operator/5
  Compare To Constant1/1 -> Logical Operator/1
  Compare To Constant2/1 -> Logical Operator/2
  Compare To Constant4/1 -> Logical Operator/3
  Compare To Constant5/1 -> Logical Operator/4
  Compare To Constant/1 -> prop2/2, prop5/1
  Logical Operator/1 -> prop1/2, not/1
  prop1/1 -> prop/1
  not/1 -> prop2/1
  prop5/1 -> prop1/1
  Compare To Constant3/1 -> prop2/3
  prop2/1 -> prop/2
  prop/1 -> prop4/1
